simulink model "untitled2"  (R2022b)
settings: Solver=ode4  StartTime=0.0  StopTime=20  FixedStep=.01  RelTol=1e-3
values from neighbouring files (symbols this model uses):
  A = exp(-a*Ts)    [RunMeFirst.m]    (also in linsys1.m = -a)
  B = 1    [RunMeFirst.m]    (also in linsys1.m = b)
  C = 1    [RunMeFirst.m]    (also in linsys1.m)
  D = 0    [RunMeFirst.m]    (also in linsys1.m)
  Qd = Q * G^2 * 1/(2*a) * (1 - exp(-2*a*Ts))    [RunMeFirst.m]
  R = .2    (= 0.2)    [RunMeFirst.m]    (also in linsys1.m = 0.5)
  Ts = .05    (= 0.05)    [RunMeFirst.m]    (also in linsys1.m = 0.1)
  x_0 = 2    [RunMeFirst.m]
  xe_0 = 3    [RunMeFirst.m]
undefined symbols (not defined in the file or in its folder): Ac, Discrete, P0, Time
libraries: ctrlSharedLib x1, dspinverses x1
settings Model: Creator=hp_desktop  LastModifiedBy=hp_desktop

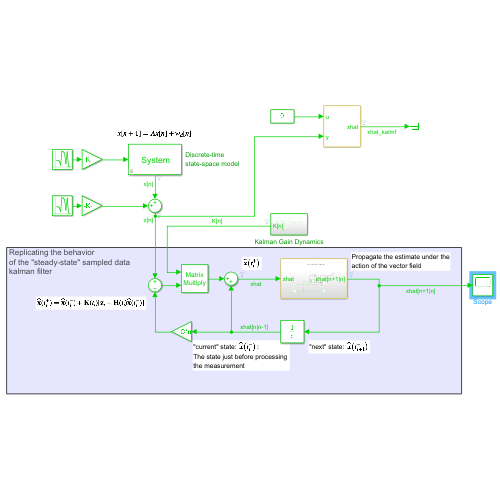
[thumbnail: Simulink's stored preview of the top-level diagram]
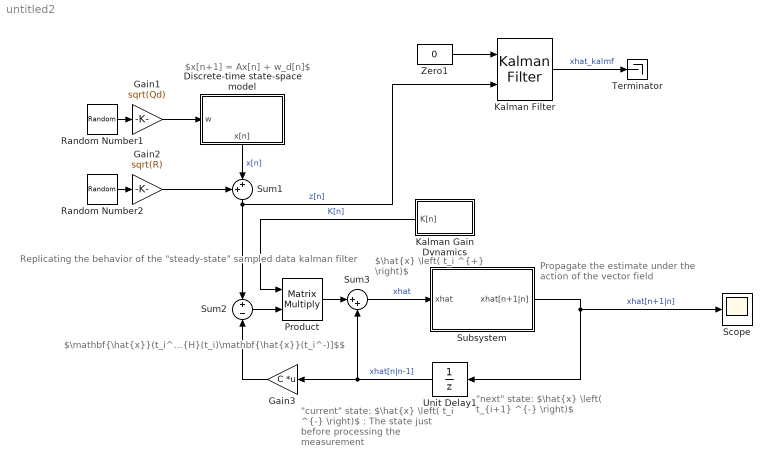
== system untitled2 ==
  note: "next" state: $\hat{x} \left( t_{i+1} ^{-} \right)$
  note: "current" state: $\hat{x} \left( t_i ^{-} \right)$ :
      | The state just before processing
      | the measurement
  note: $x[n+1] = Ax[n] + w_d[n]$
  note: $\mathbf{\hat{x}}(t_i^+)=\mathbf{\hat{x}}(t_i^-)+\mathbf{K}(t_i)[\mathbf{z}_i-\mathbf{H}(t_i)\mathbf{\hat{x}}(t_i^-)]$$
  note: Propagate the estimate under the
      | action of the vector field
  note: $\hat{x} \left( t_i ^{+} \right)$
  note: Replicating the behavior
      | of the "steady-state" sampled data
      | kalman filter
  Discrete-time state-space model : Subsystem
      settings: PortSchema="{\"entries\":[{\"content\":{\"sides\":[{\"content\":{\"connectorIds\":[\"In1\"]},\"type\":\"ConnectorPlacement.EquallySpacedRectSide\",\"uuid\":\"03aefd50-9202-4ba5-8d59-8bb562bb4022\"},{\"content\":{\"connectorIds\":[],\"side\":\"RIGHT\"},\"type\":\"ConnectorPlacement.EquallySpacedRectSide\",\"uuid\":\"1686d747-63e6-444b-902a-9e9b0bc573f1\"},{\"content\":{\"connectorIds\":[],\"side\":\"TOP\"},\"type\":\"ConnectorPlacement.EquallySpacedRectSide\",\"uuid\":\"82334134-1918-4078-909d-97976d506e34\"},{\"content\":{\"connectorIds\":[\"Out1\"],\"side\":\"BOTTOM\"},\"type\":\"ConnectorPlacement.EquallySpacedRectSide\",\"uuid\":\"6a42f511-d3ae-4f43-bbaf-a2320965212b\"}]},\"type\":\"ConnectorPlacement.EquallySpacedConnector\",\"uuid\":\"1127eaf5-13bd-4ad9-99ec-3bc039f81ae3\"}],\"packageUris\":[\"http://schema.mathworks.com/mf0/Connector/R2020b\"],\"version\":\"1.0\"}"
      mask Display: disp('\fontsize{13} System', 'texmode','on');
  Gain1 : Gain  Gain=sqrt(Qd)
  Gain2 : Gain  Gain=sqrt(R)
  Gain3 : Gain  Gain=C  Multiplication=Matrix(K*u)
  Kalman Filter : ctrlSharedLib/Kalman Filter  TimeDomain=Discrete-Time  UseCurrentEstimator=on  ModelSource=Individual A, B, C, D matrices  ModelSourceVariable=ss(0.95,1,1,0,1)  A=A  B=B  C=C  D=D  NumberOfStates=1  NumberOfInputs=1  NumberOfOutputs=1  InitialEstimateSource=Dialog  X0=xe_0  P0=10  UseK=off  UseGH=off  NumberOfProcessNoiseInputs=1  G=1  TimeInvariantG=on  H=0  TimeInvariantH=on  Q=Qd  TimeInvariantQ=on  R=R  TimeInvariantR=on  N=0  TimeInvariantN=on  AddInputPort=on  AddEnablePort=off  OutputEstimatedY=off  OutputP=off  Ts=-1
  Kalman Gain Dynamics : Subsystem
      settings: PortSchema="{\"entries\":[{\"content\":{\"sides\":[{\"content\":{\"connectorIds\":[\"Out1\"]},\"type\":\"ConnectorPlacement.EquallySpacedRectSide\",\"uuid\":\"c7f539cc-6bbb-461e-9e80-93fdf79e1c43\"},{\"content\":{\"connectorIds\":[],\"side\":\"RIGHT\"},\"type\":\"ConnectorPlacement.EquallySpacedRectSide\",\"uuid\":\"b81da1cb-7187-45ff-8ce6-2dd8ae73e17e\"},{\"content\":{\"connectorIds\":[],\"side\":\"TOP\"},\"type\":\"ConnectorPlacement.EquallySpacedRectSide\",\"uuid\":\"bbd6e24e-d46a-4248-8401-1195838f3622\"}]},\"type\":\"ConnectorPlacement.EquallySpacedConnector\",\"uuid\":\"aefde933-90b8-4e1b-866a-901b820f7ef6\"}],\"packageUris\":[\"http://schema.mathworks.com/mf0/Connector/R2020b\"],\"version\":\"1.0\"}"
  Product : Product  Multiplication=Matrix(*)
  Random Number1 : RandomNumber  SampleTime=Ts
  Random Number2 : RandomNumber  Seed=1503  SampleTime=Ts
  Scope : Scope
  Subsystem : Subsystem
  Sum1 : Sum  Inputs=++|
  Sum2 : Sum  Inputs=+-
  Sum3 : Sum  Inputs=|++
  Terminator : Terminator
  Unit Delay1 : UnitDelay  InitialCondition=xe_0  SampleTime=Ts  HasFrameUpgradeWarning=on
  Zero1 : Constant  Value=0  OutDataTypeStr=Inherit: Inherit via back propagation  SampleTime=-1
  wires:
  Gain1/1 -> Discrete-time state-space model/1(w)
  Kalman Filter/1 -> Terminator/1  "xhat_kalmf"
  Random Number1/1 -> Gain1/1
  Sum2/1 -> Product/2
  Zero1/1 -> Kalman Filter/1
  Sum1/1 -> Kalman Filter/2, Sum2/1  "z[n]"
  Gain2/1 -> Sum1/1
  Unit Delay1/1 -> Sum3/2, Gain3/1  "xhat[n|n-1]"
  Gain3/1 -> Sum2/2
  Discrete-time state-space model/1(x[n]) -> Sum1/2  "x[n]"
  Kalman Gain Dynamics/1(K[n]) -> Product/1  "K[n]"
  Product/1 -> Sum3/1
  Random Number2/1 -> Gain2/1
  Sum3/1 -> Subsystem/1(xhat)  "xhat"
  Subsystem/1(xhat[n+1|n]) -> Unit Delay1/1, Scope/1  "xhat[n+1|n]"

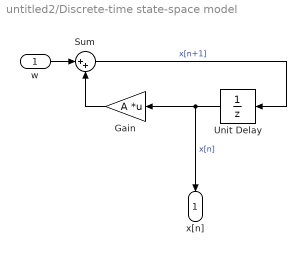
== system untitled2/Discrete-time state-space model ==
  w : Inport
  Gain : Gain  Gain=A  Multiplication=Matrix(K*u)
  Sum : Sum  Inputs=|++
  Unit Delay : UnitDelay  InitialCondition=x_0  SampleTime=Ts  HasFrameUpgradeWarning=on
  x[n] : Outport
  wires:
  Unit Delay/1 -> Gain/1, x[n]/1  "x[n]"
  Gain/1 -> Sum/2
  Sum/1 -> Unit Delay/1  "x[n+1]"
  w/1 -> Sum/1

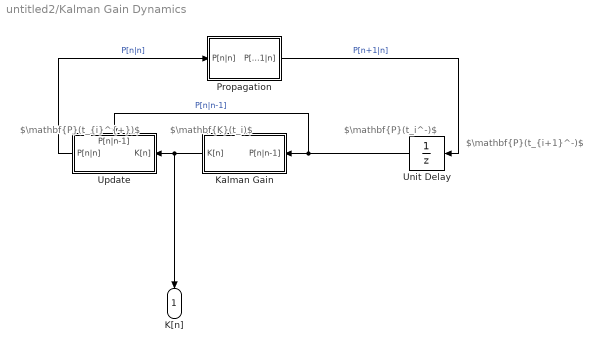
== system untitled2/Kalman Gain Dynamics ==
  note: $\mathbf{K}(t_i)$
  note: $\mathbf{P}(t_i^-)$
  note: $\mathbf{P}(t_{i+1}^-)$
  note: $\mathbf{P}(t_{i}^{+})$
  Kalman Gain : Subsystem
  Propagation : Subsystem
  Unit Delay : UnitDelay  InitialCondition=P0  SampleTime=Ts  HasFrameUpgradeWarning=on
  Update : Subsystem
      settings: PortSchema="{\"entries\":[{\"content\":{\"sides\":[{\"content\":{\"connectorIds\":[\"In1\"]},\"type\":\"ConnectorPlacement.EquallySpacedRectSide\",\"uuid\":\"7bd54a4e-5cfd-421b-8fa8-b05bee79dcff\"},{\"content\":{\"connectorIds\":[\"Out1\"],\"side\":\"RIGHT\"},\"type\":\"ConnectorPlacement.EquallySpacedRectSide\",\"uuid\":\"8559456a-1f3f-4c27-b787-d9a163f08bc3\"},{\"content\":{\"connectorIds\":[\"In2\"],\"side\":\"TOP\"},\"type\":\"ConnectorPlacement.EquallySpacedRectSide\",\"uuid\":\"58900b49-7481-44e4-9ef6-dbfb478b542d\"},{\"content\":{\"connectorIds\":[],\"side\":\"BOTTOM\"},\"type\":\"ConnectorPlacement.EquallySpacedRectSide\",\"uuid\":\"16351855-a6dc-45c4-b8fc-2d4bad2e12be\"}]},\"type\":\"ConnectorPlacement.EquallySpacedConnector\",\"uuid\":\"b6257a7b-a066-470e-8895-10173e75f3b3\"}],\"packageUris\":[\"http://schema.mathworks.com/mf0/Connector/R2020b\"],\"version\":\"1.0\"}"
  K[n] : Outport
  wires:
  Propagation/1(P[n+1|n]) -> Unit Delay/1  "P[n+1|n]"
  Unit Delay/1 -> Update/2(P[n|n-1]), Kalman Gain/1(P[n|n-1])  "P[n|n-1]"
  Kalman Gain/1(K[n]) -> K[n]/1, Update/1(K[n])
  Update/1(P[n|n]) -> Propagation/1(P[n|n])  "P[n|n]"

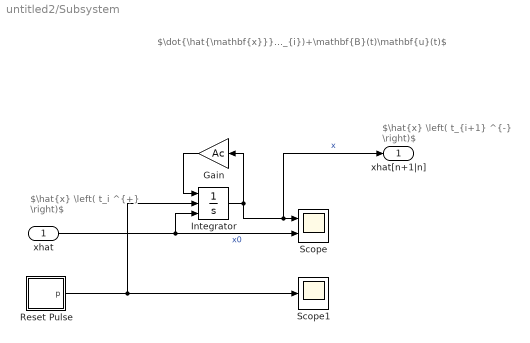
== system untitled2/Subsystem ==
  note: $\dot{\hat{\mathbf{x}}}(t/t_{i})=\mathbf{F}(t)\mathbf{\hat{x}}(t/t_{i})+\mathbf{B}(t)\mathbf{u}(t)$
  note: $\hat{x} \left( t_{i+1} ^{-} \right)$
  note: $\hat{x} \left( t_i ^{+} \right)$
  xhat : Inport
  Gain : Gain  Gain=Ac
  Integrator : Integrator  ExternalReset=either  InitialConditionSource=external
  Reset Pulse : Subsystem
  Scope : Scope  NumInputPorts=2
  Scope1 : Scope
  xhat[n+1|n] : Outport  SampleTime=Ts
  wires:
  Integrator/1 -> xhat[n+1|n]/1, Scope/1, Gain/1  "x"
  Gain/1 -> Integrator/1
  xhat/1 -> Integrator/3, Scope/2  "x0"
  Reset Pulse/1(p) -> Integrator/2, Scope1/1

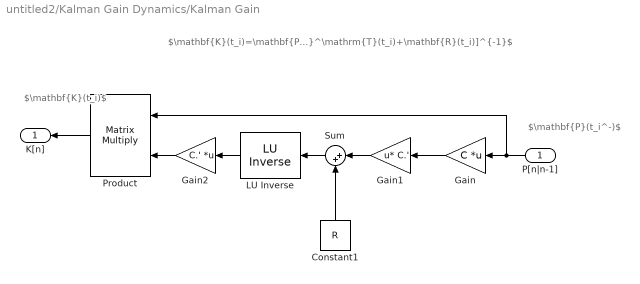
== system untitled2/Kalman Gain Dynamics/Kalman Gain ==
  note: $\mathbf{P}(t_i^-)$
  note: $\mathbf{K}(t_i)=\mathbf{P}(t_i^-)\mathbf{H}^\mathrm{T}(t_i)[\mathbf{H}(t_i)\mathbf{P}(t_i^-)\mathbf{H}^\mathrm{T}(t_i)+\mathbf{R}(t_i)]^{-1}$
  note: $\mathbf{K}(t_i)$
  P[n|n-1] : Inport
  " LU Inverse" : dspinverses/ LU Inverse
  Constant1 : Constant  Value=R  VectorParams1D=off
  Gain : Gain  Gain=C  Multiplication=Matrix(K*u)
  Gain1 : Gain  Gain=C.'  Multiplication=Matrix(u*K)
  Gain2 : Gain  Gain=C.'  Multiplication=Matrix(K*u)
  Product : Product  Multiplication=Matrix(*)
  Sum : Sum  Inputs=|++
  K[n] : Outport
  wires:
  P[n|n-1]/1 -> Product/1, Gain/1
  Gain/1 -> Gain1/1
  Gain1/1 -> Sum/1
  Constant1/1 -> Sum/2
  Sum/1 -> " LU Inverse"/1
  " LU Inverse"/1 -> Gain2/1
  Gain2/1 -> Product/2
  Product/1 -> K[n]/1

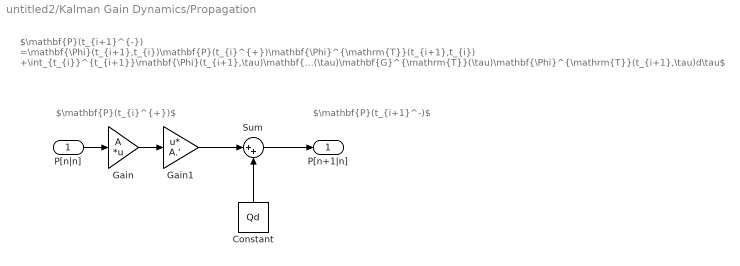
== system untitled2/Kalman Gain Dynamics/Propagation ==
  note: $\mathbf{P}(t_{i+1}^{-}) =\mathbf{\Phi}(t_{i+1},t_{i})\mathbf{P}(t_{i}^{+})\mathbf{\Phi}^{\mathrm{T}}(t_{i+1},t_{i}) +\int_{t_{i}}^{t_{i+1}}\mathbf{\Phi}(t_{i+1},\tau)\mathbf{G}(\tau)\mathbf{Q}(\tau)\mathbf{G}^{\mathrm{T}}(\tau)\mathbf{\Phi}^{\mathrm{T}}(t_{i+1},\tau)d\tau$
  note: $\mathbf{P}(t_{i}^{+})$
  note: $\mathbf{P}(t_{i+1}^-)$
  P[n|n] : Inport
  Constant : Constant  Value=Qd  VectorParams1D=off
  Gain : Gain  Gain=A  Multiplication=Matrix(K*u)
  Gain1 : Gain  Gain=A.'  Multiplication=Matrix(u*K)
  Sum : Sum  Inputs=|++
  P[n+1|n] : Outport
  wires:
  P[n|n]/1 -> Gain/1
  Gain/1 -> Gain1/1
  Gain1/1 -> Sum/1
  Constant/1 -> Sum/2
  Sum/1 -> P[n+1|n]/1

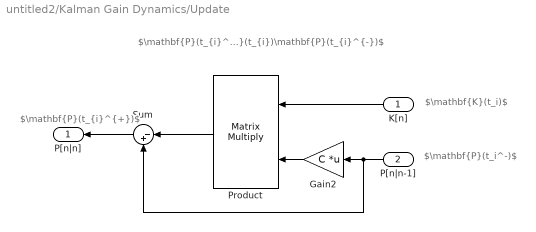
== system untitled2/Kalman Gain Dynamics/Update ==
  note: $\mathbf{P}(t_{i}^{+})$
  note: $\mathbf{P}(t_{i}^{+})=\mathbf{P}(t_{i}^{-})-\mathbf{K}(t_{i})\mathbf{H}(t_{i})\mathbf{P}(t_{i}^{-})$
  note: $\mathbf{K}(t_i)$
  note: $\mathbf{P}(t_i^-)$
  K[n] : Inport
  P[n|n-1] : Inport  Port=2
  Gain2 : Gain  Gain=C  Multiplication=Matrix(K*u)
  Product : Product  Multiplication=Matrix(*)
  Sum : Sum  Inputs=|-+
  P[n|n] : Outport
  wires:
  K[n]/1 -> Product/1
  P[n|n-1]/1 -> Sum/2, Gain2/1
  Gain2/1 -> Product/2
  Product/1 -> Sum/1
  Sum/1 -> P[n|n]/1

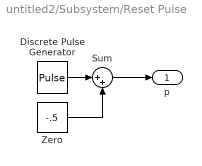
== system untitled2/Subsystem/Reset Pulse ==
  Discrete Pulse Generator : DiscretePulseGenerator  SampleTime=Ts
  Sum : Sum  Inputs=|++
  Zero : Constant  Value=-.5  OutDataTypeStr=Inherit: Inherit via back propagation
  p : Outport
  wires:
  Zero/1 -> Sum/2
  Discrete Pulse Generator/1 -> Sum/1
  Sum/1 -> p/1
